simulink model "HyL_SV_victor"  (R2013a)
settings: Solver=ode45  StartTime=0.0  StopTime=10  FixedStep=1e-3  MaxStep=0.02  MinStep=0.0005  RelTol=1e-3
model workspace (MATLAB code in the model file):
  | % Leg data
  | m1 = 1.503; % Kg
  | m2 = 0.663; % Kg
  | M = 20;     % Kg Base mass
  | 
  | l0 = 0.08;
  | l1 = 0.350; %m
  | l2 = 0.350; %m
  | l3 = 0.01;
  | 
  | lm1 = 0.1088; %m
  | lm2 = 0.1065; %m
  | I1zz = 0.02504; %kg·m2
  | I2zz = 0.0122710; %kg·m2
  | e1 = 12.7 *(pi/180); %rad
  | e2 = 0 *(pi/180); %rad
  | g  = 9.810; %m/s2
  | 
  | % ---- Lever Arm Parameters ----
  | %Hip joint
  | a1 = 0.3219;            %m
  | b1 = 0.045;             %m
  | e11 = 6.24*(pi/180);    %rad
  | e12 = 0*(pi/180);       %rad
  | 
  | %Knee joint
  | a2 = 0.3218;            %m
  | b2 = 0.045;             %m
  | e21 = 8.04*(pi/180);    %rad
  | e22 = 6*(pi/180);       %rad
  | 
  | % ----- Cylinder ------
  | c1Max = ((157 + 50 + 80) + 79)/1000; %157: fixed measure of cylinder; 50: fixed measure of load cell; 80: fixed measure of cylinder stroke; 79: chosen maximum cylinder displacement
  | c1Min = ((157 + 50 + 80) + 1)/1000; %157: fixed measure of cylinder; 50: fixed measure of load cell; 80: fixed measure of cylinder stroke; 1: chosen minimum cylinder displacement
  | 
  | % ----- Limit Angles -----
  | 
  | %Base
  | q0_0 = 1;
  | 
  | %Hip
  | q1_0 = 20*(pi/180); % Initial condition
  | 
  | Y1Max = acos((a2^2 + b2^2 - c1Max^2)/(2*a2*b2));
  | q1Max = Y1Max - e11 - e12;
  | 
  | Y1Min = acos((a2^2 + b2^2 - c1Min^2)/(2*a2*b2));
  | q1Min = Y1Min - e11 - e12;
  | % f1MinD = rad2deg(f1Min)
  | 
  | 
  | %Knee
  | q2_0 = 45*(pi/180); % Initial condition
  | 
  | Y2Max = acos((a2^2 + b2^2 - c1Max^2)/(2*a2*b2));
  | q2Max = Y2Max - e21 + e22;
  | % q2MaxD = rad2deg(q2Max)
  | 
  | Y2Min = acos((a2^2 + b2^2 - c1Min^2)/(2*a2*b2));
  | q2Min = Y2Min - e21 + e22;
  | % q2MinD = rad2deg(q2Min)
  | 
  | q0Min = l0+l1*cos(q1Min)+l2*cos(q1Min+q2Min)+l3;
undefined symbols (not defined in the file or in its folder): controllerCartSpace, Fpt, gcontact, gcPosVel, HyL_Job, referenceGenerator
libraries: simulink x3
settings Model: Creator=Toshiba  LastModifiedBy=Toshiba
settings SolverCC: ZeroCrossAlgorithm=Adaptive
settings DataIOCC: SignalLoggingSaveFormat=ModelDataLogs
settings DebuggingCC: MultiTaskDSMMsg=warning  MultiTaskCondExecSysMsg=none  StrictBusMsg=None
settings RTWCC: IncludeERTFirstTime=on

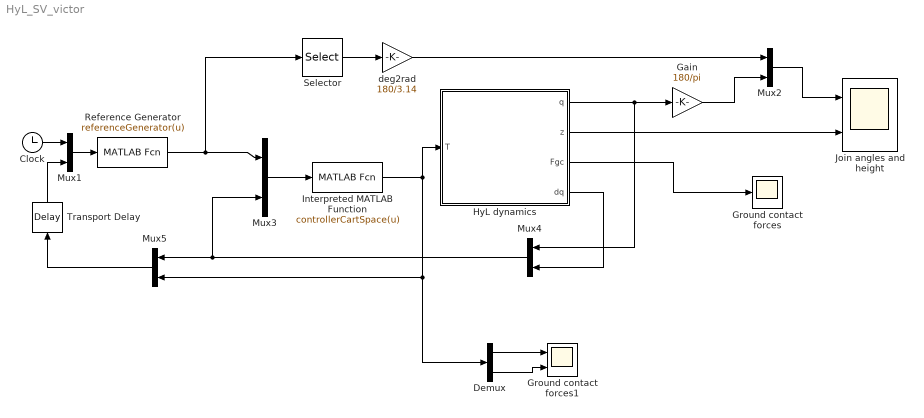
== system HyL_SV_victor ==
  Clock : Clock
  Demux : Demux  Outputs=2
  Gain : Gain  Gain=180/pi
  Ground contact forces : Scope
      settings: SaveName=ScopeData3
  Ground contact forces1 : Scope  NumInputPorts=2
      settings: YMin=-35~-25  YMax=60~175
  HyL dynamics : Subsystem
  Interpreted MATLAB Function : MATLABFcn  MATLABFcn=controllerCartSpace(u)  OutputDimensions=2
  Join angles and height : Scope  NumInputPorts=2
      settings: YMin=-150~0.275  YMax=75~0.5
  Mux{1..5} (5 alike) : Mux  Inputs=2
  Reference Generator : MATLABFcn  MATLABFcn=referenceGenerator(u)  OutputDimensions=4
  Selector : Selector  InputPortWidth=4  IndexOptions=Index vector (dialog)  Indices=[1 2]  OutputSizes=1
  Transport Delay : TransportDelay  DelayTime=0.0001
  deg2rad : Gain  Gain=180/3.14
  wires:
  HyL dynamics/1(q) -> Mux4/1, Gain/1
  HyL dynamics/2(z) -> Join angles and height/2
  Mux3/1 -> Interpreted MATLAB Function/1
  Gain/1 -> Mux2/2
  Mux2/1 -> Join angles and height/1
  HyL dynamics/3(Fgc) -> Ground contact forces/1
  HyL dynamics/4(dq) -> Mux4/2
  Interpreted MATLAB Function/1 -> Demux/1, Mux5/2, HyL dynamics/1(T)
  Reference Generator/1 -> Selector/1, Mux3/1
  Mux4/1 -> Mux5/1, Mux3/2
  Selector/1 -> deg2rad/1
  deg2rad/1 -> Mux2/1
  Mux5/1 -> Transport Delay/1
  Mux1/1 -> Reference Generator/1
  Transport Delay/1 -> Mux1/2
  Clock/1 -> Mux1/1
  Demux/1 -> Ground contact forces1/1
  Demux/2 -> Ground contact forces1/2

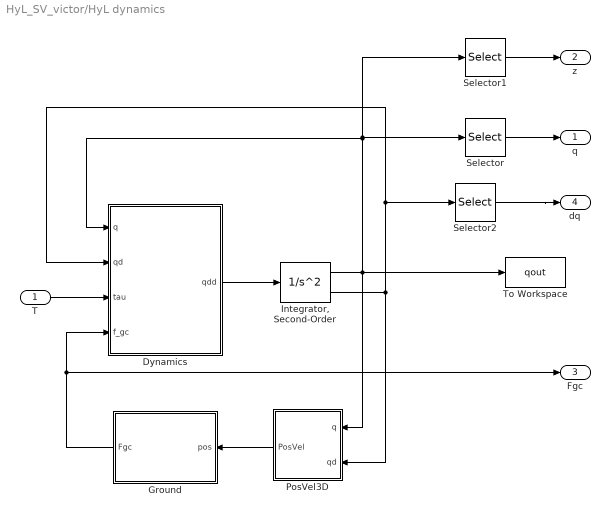
== system HyL_SV_victor/HyL dynamics ==
  T : Inport
  Dynamics : Subsystem
  Ground : Subsystem
  "Integrator, Second-Order" : SecondOrderIntegrator  ICX=[q0_0;1.16;-2.5]  LimitX=on  UpperLimitX=[inf; q1Max+10; q2Max+10]  LowerLimitX=[0; q1Min-10; q2Min-10]
  PosVel3D : Subsystem
  Selector : Selector  InputPortWidth=3  IndexOptions=Index vector (dialog)  Indices=[2 3]  OutputSizes=1
  Selector1 : Selector  InputPortWidth=3  IndexOptions=Index vector (dialog)  Indices=1  OutputSizes=1
  Selector2 : Selector  InputPortWidth=3  IndexOptions=Index vector (dialog)  Indices=[2 3]  OutputSizes=1
  To Workspace : ToWorkspace  VariableName=qout  SampleTime=-1  SaveFormat=Timeseries
  q : Outport
  z : Outport  Port=2
  Fgc : Outport  Port=3
  dq : Outport  Port=4
  wires:
  Dynamics/1(qdd) -> "Integrator, Second-Order"/1
  "Integrator, Second-Order"/1 -> Selector1/1, Selector/1, Dynamics/1(q), To Workspace/1, PosVel3D/1(q)
  "Integrator, Second-Order"/2 -> PosVel3D/2(qd), Dynamics/2(qd), Selector2/1
  Selector/1 -> q/1
  T/1 -> Dynamics/3(tau)
  Selector1/1 -> z/1
  PosVel3D/1(PosVel) -> Ground/1(pos)
  Ground/1(Fgc) -> Fgc/1, Dynamics/4(f_gc)
  Selector2/1 -> dq/1

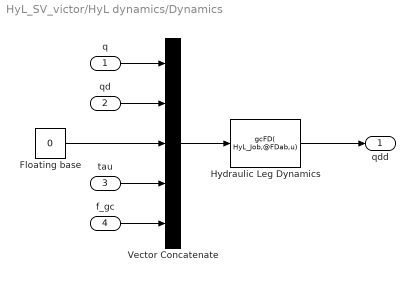
== system HyL_SV_victor/HyL dynamics/Dynamics ==
  q : Inport
  qd : Inport  Port=2
  tau : Inport  Port=3
  f_gc : Inport  Port=4
  Floating base : Constant  Value=0
  Hydraulic Leg Dynamics : MATLABFcn  MATLABFcn=gcFD( HyL_Job,@FDab,u)  OutputDimensions=[3 1]  OutputSignalType=real  Output1D=off
  Vector Concatenate : Concatenate  NumInputs=5
  qdd : Outport
  wires:
  Hydraulic Leg Dynamics/1 -> qdd/1
  Vector Concatenate/1 -> Hydraulic Leg Dynamics/1
  qd/1 -> Vector Concatenate/2
  q/1 -> Vector Concatenate/1
  f_gc/1 -> Vector Concatenate/5
  tau/1 -> Vector Concatenate/4
  Floating base/1 -> Vector Concatenate/3

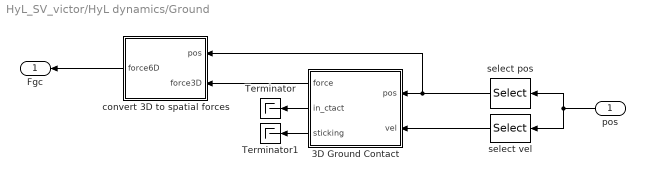
== system HyL_SV_victor/HyL dynamics/Ground ==
  pos : Inport
  3D Ground Contact : Subsystem  mask(3D Nonlinear Ground Contact with Friction){K=1e6, D=2000, mu=0.1, np=1}
      mask prompts: K "Stiffness (K)"; D "Damping (D)"; mu "Coefficient of Friction (mu)"; np "Number of Contact Points"
      mask help:
      | Given two 3xnp arrays containing contact-point positions and
      | velocities, calculate the 3xnp array of ground-reaction forces
      | acting on those points. Also calculate 1xnp boolean vectors
      | in_ctact (true if normal force >0) and sticking (true if inside
      | or on boundary of friction cone).  Zero-crossing detection is
      | enabled at both make/break contact and stick/slip transitions.
  Terminator : Terminator
  Terminator1 : Terminator
  convert 3D to spatial forces : Subsystem
  select pos : Selector  NumberOfDimensions=2  InputPortWidth=3  IndexOptions=Index vector (dialog),Select all  Indices=[1 2 3],1  OutputSizes=1,1
  select vel : Selector  NumberOfDimensions=2  InputPortWidth=3  IndexOptions=Index vector (dialog),Select all  Indices=[4 5 6],1  OutputSizes=1,1
  Fgc : Outport
  wires:
  select vel/1 -> 3D Ground Contact/2(vel)
  3D Ground Contact/1(force) -> convert 3D to spatial forces/2(force3D)
  3D Ground Contact/2(in_ctact) -> Terminator/1
  3D Ground Contact/3(sticking) -> Terminator1/1
  convert 3D to spatial forces/1(force6D) -> Fgc/1
  select pos/1 -> convert 3D to spatial forces/1(pos), 3D Ground Contact/1(pos)
  pos/1 -> select vel/1, select pos/1

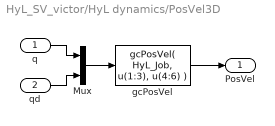
== system HyL_SV_victor/HyL dynamics/PosVel3D ==
  q : Inport
  qd : Inport  Port=2
  Mux : Mux  Inputs=2
  gcPosVel : MATLABFcn  MATLABFcn=gcPosVel( HyL_Job, u(1:3), u(4:6) )  OutputDimensions=[6 1]  OutputSignalType=real  Output1D=off
  PosVel : Outport
  wires:
  q/1 -> Mux/1
  qd/1 -> Mux/2
  Mux/1 -> gcPosVel/1
  gcPosVel/1 -> PosVel/1

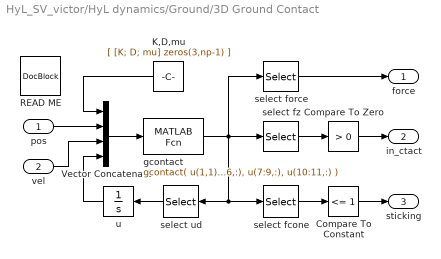
== system HyL_SV_victor/HyL dynamics/Ground/3D Ground Contact ==
  pos : Inport
  vel : Inport  Port=2
  Compare To Constant : simulink/Logic and Bit Operations/Compare To Constant  relop=<=  const=1  OutDataTypeStr=boolean
  Compare To Zero : simulink/Logic and Bit Operations/Compare To Zero  relop=>  OutDataTypeStr=boolean
  K,D,mu : Constant  Value=[ [K; D; mu] zeros(3,np-1) ]  VectorParams1D=off
  READ ME : simulink/Model-Wide Utilities/DocBlock  DocumentType=Text
      content=|
      | The constant block supplies the parameters K, D and mu to the function
      | gcontact.  This is necessary because K, D and mu are defined in the
      | workspace of this particular masked subsystem, but the executable
      | expression in the "MATLAB Function" block does not have access to this
      | workspace, so the symbols K, D and mu cannot appear directly in the
      | executable expression.
      |
      | The ">0" block and the "<=1" block both have zero-crossing enabled.  The
      | former detects transitions between contact and non-contact, whereas the
      | latter detects transitions between sticking (due to friction) and
      | slipping.  A point can be sticking only if it is also in contact.  A
      | zero-crossing event occurs whenever any one point makes a transition.
      |
      | The state variable, u, is a 2x(np) matrix containing the horizontal
      | component of the local ground deformation for each point.  This quantity
      | is used to calculate the tangential (i.e., frictional) component of the
      | ground reaction force.
      |
      | When a point loses contact, its associated state variable, u(:,i), decays
      | to zero with a time constant of D/K.  If this ratio is small then the
      | corresponding differential equation is fast, and it is necessary to use
      | small integration time steps.  For example, if K=1e6 and D=2000 then
      | D/K=0.002 and u(:,i) decays in proportion to exp(-500t).  Increasing K
      | makes the surface stiffer, and decreasing D/K makes it bouncier, but the
      | latter also makes the post-contact recovery faster.  The degree of
      | bounciness depends on the mass of the impacting body: a heavier body will
      | bounce more.
      |
      | To adapt this subsystem to work in 2D, the only things that change are the
      | row dimensions of various matrices.  You will have to alter the row
      | selections in the executable expression in the "MATLAB Function" block,
      | and also the dimensions of its output matrix, and you will have to change
      | the row selections in the various "select" blocks.
      |
      | For more information, see "The Simulink Ground Contact Model" in the
      | spatial_v2 documentation directory.
  Vector Concatenate : Concatenate  NumInputs=4  Mode=Multidimensional array
  gcontact : MATLABFcn  MATLABFcn=gcontact( u(1,1), u(2,1), u(3,1), u(4:6,:), u(7:9,:), u(10:11,:) )  OutputDimensions=[6 np]  OutputSignalType=real  Output1D=off
  select fcone : Selector  NumberOfDimensions=2  InputPortWidth=3  IndexOptions=Index vector (dialog),Select all  Indices=[6],1  OutputSizes=1,1
  select force : Selector  NumberOfDimensions=2  InputPortWidth=3  IndexOptions=Index vector (dialog),Select all  Indices=[1 2 3],1  OutputSizes=1,1
  select fz : Selector  NumberOfDimensions=2  InputPortWidth=3  IndexOptions=Index vector (dialog),Select all  Indices=[3],1  OutputSizes=1,1
  select ud : Selector  NumberOfDimensions=2  InputPortWidth=3  IndexOptions=Index vector (dialog),Select all  Indices=[4 5],1  OutputSizes=1,1
  u : Integrator
  force : Outport
  in_ctact : Outport  Port=2
  sticking : Outport  Port=3
  wires:
  Vector Concatenate/1 -> gcontact/1
  select ud/1 -> u/1
  gcontact/1 -> select fz/1, select ud/1, select fcone/1, select force/1
  select force/1 -> force/1
  select fz/1 -> Compare To Zero/1
  Compare To Zero/1 -> in_ctact/1
  select fcone/1 -> Compare To Constant/1
  Compare To Constant/1 -> sticking/1
  u/1 -> Vector Concatenate/4
  vel/1 -> Vector Concatenate/3
  pos/1 -> Vector Concatenate/2
  K,D,mu/1 -> Vector Concatenate/1

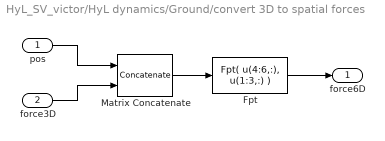
== system HyL_SV_victor/HyL dynamics/Ground/convert 3D to spatial forces ==
  pos : Inport
  force3D : Inport  Port=2
  Fpt : MATLABFcn  MATLABFcn=Fpt( u(4:6,:), u(1:3,:) )  OutputSignalType=real  Output1D=off
  Matrix Concatenate : Concatenate  Mode=Multidimensional array
  force6D : Outport
  wires:
  force3D/1 -> Matrix Concatenate/2
  pos/1 -> Matrix Concatenate/1
  Matrix Concatenate/1 -> Fpt/1
  Fpt/1 -> force6D/1
